simulink model "non_unity_gain_feedback"  (Simulink 8.7)
settings: Solver=ode45  StartTime=0.0  StopTime=500  RelTol=1e-3
settings Model: Creator=eechris  LastModifiedBy=eechris
settings DataIOCC: SignalLoggingSaveFormat=ModelDataLogs
settings OptimizationCC: ExpressionDepthLimit=2147483647
settings DebuggingCC: SolverPrmCheckMsg=warning  FcnCallInpInsideContextMsg=UseLocalSettings  StateNameClashWarn=warning
settings GRTTargetCC: CombineOutputUpdateFcns=off  GRTInterface=on

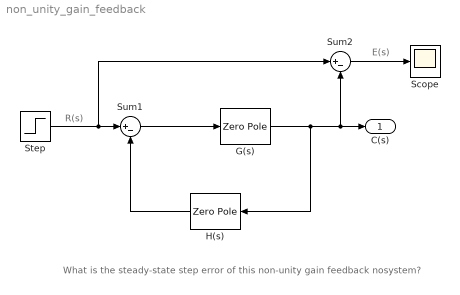
== system non_unity_gain_feedback ==
  note: R(s)
  note: E(s)
  note: What is the steady-state step error of this non-unity gain feedback nosystem?
  G(s) : ZeroPole  Zeros=[]  Poles=[0 -10]  Gain=1
  H(s) : ZeroPole  Zeros=[]  Poles=[-5]  Gain=1
  Scope : Scope
  Step : Step  Time=0  SampleTime=0
  Sum1 : Sum  Inputs=|+-
  Sum2 : Sum  Inputs=|+-
  C(s) : Outport
  wires:
  G(s)/1 -> Sum2/2, C(s)/1, H(s)/1
  Step/1 -> Sum2/1, Sum1/1
  Sum1/1 -> G(s)/1
  H(s)/1 -> Sum1/2
  Sum2/1 -> Scope/1
